simulink library "INT_ASMod_TempCatMod"  (R2016b)
settings: Solver=VariableStepAuto  StartTime=0.0  StopTime=10.0  RelTol=1e-3
settings Model: Creator=Administrator  LastModifiedBy=Administrator

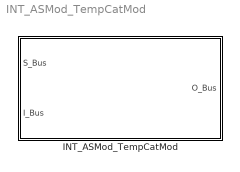
== system INT_ASMod_TempCatMod ==
  INT_ASMod_TempCatMod : Subsystem

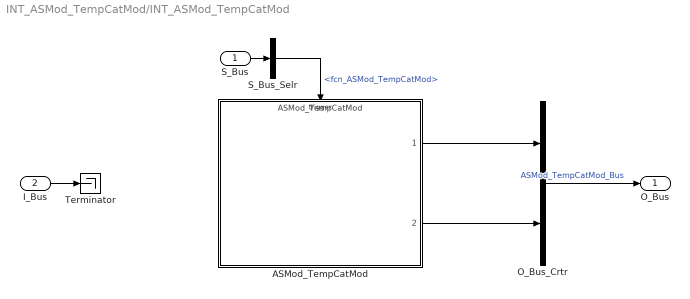
== system INT_ASMod_TempCatMod/INT_ASMod_TempCatMod ==
  S_Bus : Inport
  I_Bus : Inport  Port=2
  ASMod_TempCatMod : ModelReference  ModelNameDialog=ASMod_TempCatMod  SimulationMode=Normal  ModelReferenceVersion=1.3  TriggerPortName=function  TriggerPortTriggerType=function-call  TriggerPortStatesWhenEnabling=held
  O_Bus_Crtr : BusCreator  Inputs=2
  S_Bus_Selr : BusSelector  OutputSignals=fcn_ASMod_TempCatMod
  Terminator : Terminator
  O_Bus : Outport
  wires:
  S_Bus_Selr/1 -> ASMod_TempCatMod/Trigger  "<fcn_ASMod_TempCatMod>"
  S_Bus/1 -> S_Bus_Selr/1
  I_Bus/1 -> Terminator/1
  O_Bus_Crtr/1 -> O_Bus/1  "ASMod_TempCatMod_Bus"
  ASMod_TempCatMod/1 -> O_Bus_Crtr/1
  ASMod_TempCatMod/2 -> O_Bus_Crtr/2
